simulink model "hexapod"  (R2022a)
settings: Solver=ode2  StartTime=0.0  StopTime=10.0  FixedStep=1e-4  RelTol=1e-3  AbsTol=1e-3  EnableMultiTasking=on
values from neighbouring files (symbols this model uses):
  N = 2    [gen_singleGait.m]
  s = t/T    [gait_mv_backward.m]    (also in gait_mv_forward.m; gait_mv_left.m; gait_mv_right.m; gait_rot_clockwise.m)
undefined symbols (not defined in the file or in its folder): X, Y, Z
libraries: sm_lib x90, nesl_utility x19, Contact_Forces_Lib x6, simulink x1
(part 1 of 4)
settings Model: Creator=world  LastModifiedBy=world
settings SolverCC: AutoScaleAbsTol=off  AlgebraicLoopSolver=TrustRegion  MaxZcPerStep=1
settings DataIOCC: LimitDataPoints=on  MaxDataPoints=10000
settings OptimizationCC: LifeSpan=inf
settings DebuggingCC: UnconnectedInputMsg=warning  UnconnectedOutputMsg=warning  UnconnectedLineMsg=warning  AllowSymbolicDim=off  SFUnexpectedBacktrackingDiag=warning  SFNoUnconditionalDefaultTransitionDiag=warning  SFExecutionAtInitializationDiag=none  SFMachineParentedDataDiag=warning  ArithmeticOperatorsInVariantConditions=warning
settings SFSimCC: SimUseLocalCustomCode=off  CustomCodeUndefinedFunction=UseInterfaceOnly
settings RTWCC: RTWUseLocalCustomCode=off  DLArmComputeVersion=19.05
settings CodeAppCC: StateflowObjectComments=on
settings GRTTargetCC: TargetLangStandard=C89/C90 (ANSI)
settings ConfigComp: CovMetricSettings=dw  CovSaveCumulativeToWorkspaceVar=on  CovSaveSingleToWorkspaceVar=on  CovExternalEMLEnable=off  CovSFcnEnable=off
settings SimscapeCC: SimscapeLogType=all  SimscapeLogSimulationStatistics=on  SimscapeLogDataHistory=10000
settings DiagnosticsConfigSet: SimMechanicsRigidlyBoundBlock=warning

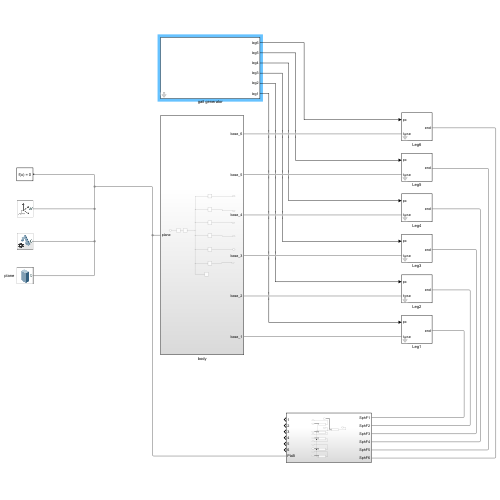
[thumbnail: Simulink's stored preview of the top-level diagram]
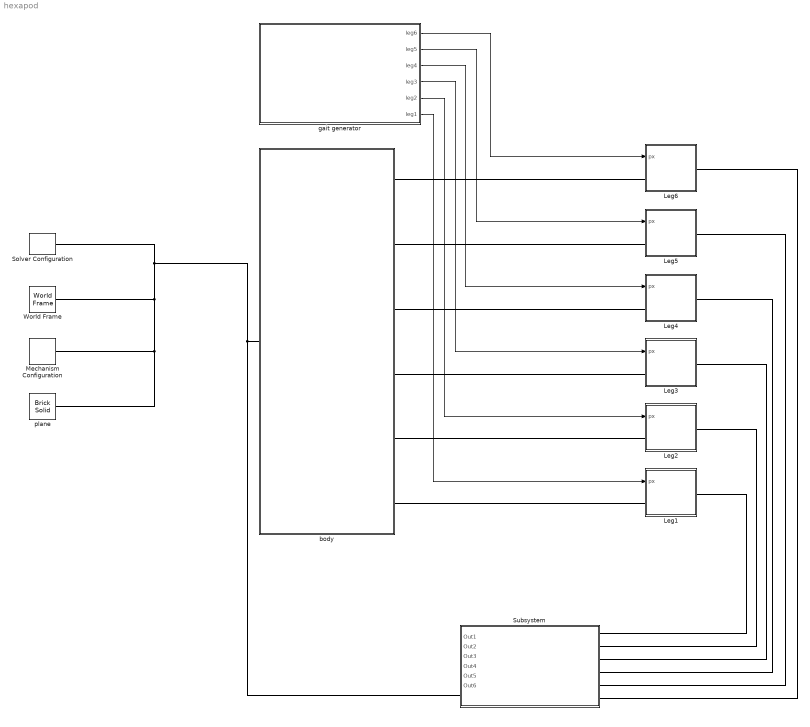
== system hexapod ==
  Leg1 : Subsystem  mask{LegNumber=1, theta1=80, theta2=90, theta3=100, l1=45, l2=93.5, l3=124.14, xx1=115, yy1=65, yy2=95}
      mask prompts: LegNumber "腿号"
      mask DialogControl ParameterGroupVar Prompt: 参数
  Leg2 : Subsystem  mask{LegNumber=2, theta1=80, theta2=90, theta3=100, l1=45, l2=93.5, l3=124.14, xx1=115, yy1=65, yy2=95}
      mask prompts: LegNumber "腿号"
      mask DialogControl ParameterGroupVar Prompt: 参数
  Leg3 : Subsystem  mask{LegNumber=3, theta1=80, theta2=90, theta3=100, l1=45, l2=93.5, l3=124.14, xx1=115, yy1=65, yy2=95}
      mask prompts: LegNumber "腿号"
      mask DialogControl ParameterGroupVar Prompt: 参数
  Leg4 : Subsystem  mask{LegNumber=4, theta1=80, theta2=90, theta3=100, l1=45, l2=93.5, l3=124.14, xx1=115, yy1=65, yy2=95}
      mask prompts: LegNumber "腿号"
      mask DialogControl ParameterGroupVar Prompt: 参数
  Leg5 : Subsystem  mask{LegNumber=5, theta1=80, theta2=90, theta3=100, l1=45, l2=93.5, l3=124.14, xx1=115, yy1=65, yy2=95}
      mask prompts: LegNumber "腿号"
      mask DialogControl ParameterGroupVar Prompt: 参数
  Leg6 : Subsystem  mask{LegNumber=6, theta1=80, theta2=90, theta3=100, l1=45, l2=93.5, l3=124.14, xx1=115, yy1=65, yy2=95}
      mask prompts: LegNumber "腿号"
      mask DialogControl ParameterGroupVar Prompt: 关键参数
      mask DialogControl Container4 Prompt: 几何参数
  Mechanism Configuration : sm_lib/Utilities/Mechanism Configuration  UniformGravity=Constant  GravityVector=[0 0 -9.80665]  GravityUnits=m/s^2  LinearizationDelta=0.001  JointModeTransitionNonlinearIterations=2
  Solver Configuration : nesl_utility/Solver Configuration  PhysicalDomain=network_engine_domain  SubClassName=solver  LeftPortType=input  RightPortType=generic  Tones=[]  Harmonics=[]  SimulateNoise=off  Profile=off  UseLocalSampling=off  EnableSwitchedLinearOptims=on  FrequencyDomain=off  UseCCode=off  RelTol=0.001  AbsTol=1e-06  MinStep=1e-09  ToWorkspace=off  RevertToSquareIcSolve=off  NumHomotopyIterations=100  PhasorMode=off  PhasorModeNumHarmonics=1  IndexReductionMethod=DerivativeReplacement  DoDC=off  ResidualTolerance=1e-09  UseLocalSolver=off  LocalSolverChoice=NE_BACKWARD_EULER_ADVANCER  LocalSolverSampleTime=0.001  DoFixedCost=off  MaxNonlinIter=3  MaxModeIter=2  ComputeImpulses=off  ImpulseIterations=2  LinearAlgebra=Sparse  LinearAlgebraNumThread=0  EquationFormulation=NE_TIME_EF  DelaysMemoryBudget=1024  AutomaticFiltering=on  FilteringTimeConstant=0.001  PartitionStorageMethod=AS_NEEDED  PartitionMemoryBudget=1024  PartitionMethod=FAST
      settings: SourceProductBaseCode=SS,PW,VE
  Subsystem : Subsystem
  World Frame : sm_lib/Frames and Transforms/World Frame
  body : Subsystem
  gait generator : Subsystem  mask{mode=high position, action=rotate clockwise, LL=2*50, AAng=45, HH=60, xx1=115, yy1=65, yy2=95, theta1=80, theta2=90, theta3=100, xxx1=[136.27,142.15], yyy1=[191.37,224.71], yyy2=[233.14,257], zzz1=[-67.38,-118]}
      mask TypeOptions mode: low position | high position
      mask TypeOptions action: move forward | move backward | move left | move right | rotate counterclockwise | rotate clockwise
      mask DialogControl Container6 Prompt: modification
      mask DialogControl Container7 Prompt: parameter
      mask DialogControl Container8 Prompt: gait parameter
      mask DialogControl Container5 Prompt: mechanical configuration
  plane : sm_lib/Body Elements/Brick Solid  GraphicAmbientColor=[0.15 0.15 0.15 1.0]  BasedOnType=Density  BrickDimensions=[5000 5000 1]  BrickDimensionUnits=mm  CenterOfMass=[0 0 0]  CenterOfMassUnits=m  GraphicDiffuseColor=[0.5 0.5 0.5]  Density=1000  DensityUnits=kg/m^3  DoExposeReferenceFrame=on  GraphicEmissiveColor=[0.0 0.0 0.0 1.0]  ExportEntireGeometry=off  SerializedFrames=<Frames/>  MarkerShape=Sphere  MarkerSize=10  GraphicType=FromGeometry  InertiaType=CalculateFromGeometry  Mass=1  MassUnits=kg  MomentsOfInertia=[1 1 1]  MomentsOfInertiaUnits=kg*m^2  GraphicOpacity=1.0  ProductsOfInertia=[0 0 0]  ProductsOfInertiaUnits=kg*m^2  GraphicShininess=75  GraphicSpecularColor=[0.5 0.5 0.5 1.0]  GraphicVisPropType=SimpleVisualProperties
  wires:
  gait generator/1(leg6) -> Leg6/1(px)
  gait generator/2(leg5) -> Leg5/1(px)
  gait generator/3(leg4) -> Leg4/1(px)
  gait generator/4(leg3) -> Leg3/1(px)
  gait generator/5(leg2) -> Leg2/1(px)
  gait generator/6(leg1) -> Leg1/1(px)
  connections:
  plane/RConn1 -- Mechanism Configuration/RConn1 -- World Frame/RConn1 -- Solver Configuration/RConn1 -- Subsystem/RConn1 -- body/LConn1
  Leg2/RConn1 -- Subsystem/LConn2
  Leg3/RConn1 -- Subsystem/LConn3
  Subsystem/LConn4 -- Leg4/RConn1
  Leg5/RConn1 -- Subsystem/LConn5
  Subsystem/LConn6 -- Leg6/RConn1
  Leg1/LConn1 -- body/RConn6
  Leg1/RConn1 -- Subsystem/LConn1
  body/RConn5 -- Leg2/LConn1
  body/RConn4 -- Leg3/LConn1
  body/RConn3 -- Leg4/LConn1
  Leg5/LConn1 -- body/RConn2
  body/RConn1 -- Leg6/LConn1

== system hexapod/Leg1 ==
  px : Inport
  Constant : Constant  Value=theta1
  Constant1 : Constant  Value=theta2
  Constant2 : Constant  Value=theta3
  Constant3 : Constant  Value=l1
  Constant4 : Constant  Value=l2
  Constant5 : Constant  Value=l3
  Constant6 : Constant  Value=xx1
  Constant7 : Constant  Value=yy1
  Constant8 : Constant  Value=yy2
  Demux : Demux  Outputs=3
  leg1 : Subsystem
  w-leg1 : Subsystem
  base : PMIOPort  Side=Left
  end : PMIOPort  Port=2  Side=Right
  wires:
  Constant8/1 -> w-leg1/12(yy2)
  Constant7/1 -> w-leg1/11(yy1)
  Constant6/1 -> w-leg1/10(xx1)
  Constant/1 -> w-leg1/4(theta1)
  Constant1/1 -> w-leg1/5(theta2)
  Constant2/1 -> w-leg1/6(theta3)
  Constant3/1 -> w-leg1/7(l1)
  Constant4/1 -> w-leg1/8(l2)
  Constant5/1 -> w-leg1/9(l3)
  Demux/1 -> w-leg1/1(x0)
  Demux/2 -> w-leg1/2(y0)
  Demux/3 -> w-leg1/3(z0)
  px/1 -> Demux/1
  connections:
  base/RConn1 -- leg1/LConn1
  leg1/RConn1 -- end/RConn1
  w-leg1/RConn3 -- leg1/LConn4
  leg1/LConn2 -- w-leg1/RConn1
  w-leg1/RConn2 -- leg1/LConn3

== system hexapod/Leg2 ==
  px : Inport
  Constant : Constant  Value=theta1
  Constant1 : Constant  Value=theta2
  Constant2 : Constant  Value=theta3
  Constant3 : Constant  Value=l1
  Constant4 : Constant  Value=l2
  Constant5 : Constant  Value=l3
  Constant6 : Constant  Value=xx1
  Constant7 : Constant  Value=yy1
  Constant8 : Constant  Value=yy2
  Demux : Demux  Outputs=3
  leg1 : Subsystem
  w-leg1 : Subsystem
  base : PMIOPort  Side=Left
  end : PMIOPort  Port=2  Side=Right
  wires:
  px/1 -> Demux/1
  Demux/3 -> w-leg1/3(z0)
  Demux/2 -> w-leg1/2(y0)
  Demux/1 -> w-leg1/1(x0)
  Constant5/1 -> w-leg1/9(l3)
  Constant4/1 -> w-leg1/8(l2)
  Constant3/1 -> w-leg1/7(l1)
  Constant2/1 -> w-leg1/6(theta3)
  Constant1/1 -> w-leg1/5(theta2)
  Constant/1 -> w-leg1/4(theta1)
  Constant6/1 -> w-leg1/10(xx1)
  Constant7/1 -> w-leg1/11(yy1)
  Constant8/1 -> w-leg1/12(yy2)
  connections:
  w-leg1/RConn2 -- leg1/LConn3
  leg1/LConn2 -- w-leg1/RConn1
  w-leg1/RConn3 -- leg1/LConn4
  leg1/RConn1 -- end/RConn1
  base/RConn1 -- leg1/LConn1

== system hexapod/Leg3 ==
  px : Inport
  Constant : Constant  Value=theta1
  Constant1 : Constant  Value=theta2
  Constant2 : Constant  Value=theta3
  Constant3 : Constant  Value=l1
  Constant4 : Constant  Value=l2
  Constant5 : Constant  Value=l3
  Constant6 : Constant  Value=xx1
  Constant7 : Constant  Value=yy1
  Constant8 : Constant  Value=yy2
  Demux : Demux  Outputs=3
  leg1 : Subsystem
  w-leg1 : Subsystem
  base : PMIOPort  Side=Left
  end : PMIOPort  Port=2  Side=Right
  wires:
  Constant8/1 -> w-leg1/12(yy2)
  Constant7/1 -> w-leg1/11(yy1)
  Constant6/1 -> w-leg1/10(xx1)
  Constant/1 -> w-leg1/4(theta1)
  Constant1/1 -> w-leg1/5(theta2)
  Constant2/1 -> w-leg1/6(theta3)
  Constant3/1 -> w-leg1/7(l1)
  Constant4/1 -> w-leg1/8(l2)
  Constant5/1 -> w-leg1/9(l3)
  Demux/1 -> w-leg1/1(x0)
  Demux/2 -> w-leg1/2(y0)
  Demux/3 -> w-leg1/3(z0)
  px/1 -> Demux/1
  connections:
  base/RConn1 -- leg1/LConn1
  leg1/RConn1 -- end/RConn1
  w-leg1/RConn3 -- leg1/LConn4
  leg1/LConn2 -- w-leg1/RConn1
  w-leg1/RConn2 -- leg1/LConn3

== system hexapod/Leg4 ==
  px : Inport
  Constant : Constant  Value=theta1
  Constant1 : Constant  Value=theta2
  Constant2 : Constant  Value=theta3
  Constant3 : Constant  Value=l1
  Constant4 : Constant  Value=l2
  Constant5 : Constant  Value=l3
  Constant6 : Constant  Value=xx1
  Constant7 : Constant  Value=yy1
  Constant8 : Constant  Value=yy2
  Demux : Demux  Outputs=3
  leg1 : Subsystem
  w-leg1 : Subsystem
  base : PMIOPort  Side=Left
  end : PMIOPort  Port=2  Side=Right
  wires:
  px/1 -> Demux/1
  Demux/3 -> w-leg1/3(z0)
  Demux/2 -> w-leg1/2(y0)
  Demux/1 -> w-leg1/1(x0)
  Constant5/1 -> w-leg1/9(l3)
  Constant4/1 -> w-leg1/8(l2)
  Constant3/1 -> w-leg1/7(l1)
  Constant2/1 -> w-leg1/6(theta3)
  Constant1/1 -> w-leg1/5(theta2)
  Constant/1 -> w-leg1/4(theta1)
  Constant6/1 -> w-leg1/10(xx1)
  Constant7/1 -> w-leg1/11(yy1)
  Constant8/1 -> w-leg1/12(yy2)
  connections:
  w-leg1/RConn2 -- leg1/LConn3
  leg1/LConn2 -- w-leg1/RConn1
  w-leg1/RConn3 -- leg1/LConn4
  leg1/RConn1 -- end/RConn1
  base/RConn1 -- leg1/LConn1

== system hexapod/Leg5 ==
  px : Inport
  Constant : Constant  Value=theta1
  Constant1 : Constant  Value=theta2
  Constant2 : Constant  Value=theta3
  Constant3 : Constant  Value=l1
  Constant4 : Constant  Value=l2
  Constant5 : Constant  Value=l3
  Constant6 : Constant  Value=xx1
  Constant7 : Constant  Value=yy1
  Constant8 : Constant  Value=yy2
  Demux : Demux  Outputs=3
  leg1 : Subsystem
  w-leg1 : Subsystem
  base : PMIOPort  Side=Left
  end : PMIOPort  Port=2  Side=Right
  wires:
  Constant8/1 -> w-leg1/12(yy2)
  Constant7/1 -> w-leg1/11(yy1)
  Constant6/1 -> w-leg1/10(xx1)
  Constant/1 -> w-leg1/4(theta1)
  Constant1/1 -> w-leg1/5(theta2)
  Constant2/1 -> w-leg1/6(theta3)
  Constant3/1 -> w-leg1/7(l1)
  Constant4/1 -> w-leg1/8(l2)
  Constant5/1 -> w-leg1/9(l3)
  Demux/1 -> w-leg1/1(x0)
  Demux/2 -> w-leg1/2(y0)
  Demux/3 -> w-leg1/3(z0)
  px/1 -> Demux/1
  connections:
  base/RConn1 -- leg1/LConn1
  leg1/RConn1 -- end/RConn1
  w-leg1/RConn3 -- leg1/LConn4
  leg1/LConn2 -- w-leg1/RConn1
  w-leg1/RConn2 -- leg1/LConn3

== system hexapod/Leg6 ==
  note: w-leg1
  px : Inport
  Constant : Constant  Value=theta1
  Constant1 : Constant  Value=theta2
  Constant2 : Constant  Value=theta3
  Constant3 : Constant  Value=l1
  Constant4 : Constant  Value=l2
  Constant5 : Constant  Value=l3
  Constant6 : Constant  Value=xx1
  Constant7 : Constant  Value=yy1
  Constant8 : Constant  Value=yy2
  Constant9 : Constant  Value=LegNumber
  Demux : Demux  Outputs=3
  MATLAB Function : MATLAB Function  TreatAsAtomicUnit=on
  Scope : Scope  NumInputPorts=3
  Scope1 : Scope  NumInputPorts=3
  Simulink-PS Converter : nesl_utility/Simulink-PS Converter  PhysicalDomain=network_engine_domain  SubClassName=ps_input  LeftPortType=input  RightPortType=output  PseudoPeriodic=off  Frequencies=[]  NoiseDistribution=none  NoiseParameters=[]  Unit=1  AffineConversion=off  FilteringAndDerivatives=filter  SimscapeFilterOrder=2  InputFilterTimeConstant=0.001  UdotUserProvided=0
      settings: SourceProductBaseCode=SS,PW,VE
  Simulink-PS Converter1 : nesl_utility/Simulink-PS Converter  PhysicalDomain=network_engine_domain  SubClassName=ps_input  LeftPortType=input  RightPortType=output  PseudoPeriodic=off  Frequencies=[]  NoiseDistribution=none  NoiseParameters=[]  Unit=1  AffineConversion=off  FilteringAndDerivatives=filter  SimscapeFilterOrder=2  InputFilterTimeConstant=0.001  UdotUserProvided=0
      settings: SourceProductBaseCode=SS,PW,VE
  Simulink-PS Converter2 : nesl_utility/Simulink-PS Converter  PhysicalDomain=network_engine_domain  SubClassName=ps_input  LeftPortType=input  RightPortType=output  PseudoPeriodic=off  Frequencies=[]  NoiseDistribution=none  NoiseParameters=[]  Unit=1  AffineConversion=off  FilteringAndDerivatives=filter  SimscapeFilterOrder=2  InputFilterTimeConstant=0.001  UdotUserProvided=0
      settings: SourceProductBaseCode=SS,PW,VE
  leg1 : Subsystem
  base : PMIOPort  Side=Left
  end : PMIOPort  Port=2  Side=Right
  wires:
  MATLAB Function/3(ang3) -> Simulink-PS Converter2/1, Scope/3
  px/1 -> Demux/1
  Demux/2 -> Scope1/2, MATLAB Function/3(y0)
  Demux/3 -> Scope1/3, MATLAB Function/4(z0)
  Demux/1 -> Scope1/1, MATLAB Function/2(x0)
  Constant9/1 -> MATLAB Function/1(i)
  MATLAB Function/2(ang2) -> Scope/2, Simulink-PS Converter1/1
  MATLAB Function/1(ang1) -> Scope/1, Simulink-PS Converter/1
  Constant2/1 -> MATLAB Function/7(theta3)
  Constant/1 -> MATLAB Function/5(theta1)
  Constant5/1 -> MATLAB Function/10(l3)
  Constant4/1 -> MATLAB Function/9(l2)
  Constant3/1 -> MATLAB Function/8(l1)
  Constant1/1 -> MATLAB Function/6(theta2)
  Constant6/1 -> MATLAB Function/11(xx1)
  Constant7/1 -> MATLAB Function/12(yy1)
  Constant8/1 -> MATLAB Function/13(yy2)
  connections:
  base/RConn1 -- leg1/LConn1
  leg1/RConn1 -- end/RConn1
  Simulink-PS Converter2/RConn1 -- leg1/LConn4
  Simulink-PS Converter/RConn1 -- leg1/LConn2
  Simulink-PS Converter1/RConn1 -- leg1/LConn3

== system hexapod/Subsystem ==
  Sphere to Plane Force{,1..5} (6 alike) : Contact_Forces_Lib/3D/Sphere to Plane Force  sphere_rad=0.01  plane_lenx=5  plane_leny=5  plane_depth=0.01  force_law=Linear  k_contact=1e7  b_contact=1e3  pen_full_damp_F=1e-4  pen_exponent=1  custom_param_1=1  custom_param_2=1  friction_law=Stick-Slip Continuous  mu_kinetic=0.5  mu_static=0.7  v_thr=0.001  vis_on=on  vis_opc_en=0  vis_len_plaBz=0.005  vis_clr=[0.9 0.2 0.2]  vis_opc=0.7
  SphF1 : PMIOPort  Side=Left
  SphF2 : PMIOPort  Port=2  Side=Left
  SphF3 : PMIOPort  Port=3  Side=Left
  PlaB : PMIOPort  Port=4  Side=Right
  SphF4 : PMIOPort  Port=5  Side=Left
  SphF5 : PMIOPort  Port=6  Side=Left
  SphF6 : PMIOPort  Port=7  Side=Left
  Out1 : Outport
  Out2 : Outport  Port=2
  Out3 : Outport  Port=3
  Out4 : Outport  Port=4
  Out5 : Outport  Port=5
  Out6 : Outport  Port=6
  wires:
  Sphere to Plane Force3/1 -> Out4/1
  Sphere to Plane Force1/1 -> Out2/1
  Sphere to Plane Force4/1 -> Out5/1
  Sphere to Plane Force5/1 -> Out6/1
  Sphere to Plane Force2/1 -> Out3/1
  Sphere to Plane Force/1 -> Out1/1
  connections:
  SphF3/RConn1 -- Sphere to Plane Force3/LConn1
  SphF1/RConn1 -- Sphere to Plane Force5/LConn1
  SphF4/RConn1 -- Sphere to Plane Force2/LConn1
  SphF2/RConn1 -- Sphere to Plane Force4/LConn1
  Sphere to Plane Force5/RConn1 -- Sphere to Plane Force/RConn1 -- Sphere to Plane Force3/RConn1 -- Sphere to Plane Force4/RConn1 -- Sphere to Plane Force2/RConn1 -- Sphere to Plane Force1/RConn1 -- PlaB/RConn1
  Sphere to Plane Force/LConn1 -- SphF6/RConn1
  SphF5/RConn1 -- Sphere to Plane Force1/LConn1

== system hexapod/body ==
  6-DOF Joint : sm_lib/Joints/6-DOF Joint  JointMode=Normal  SenseConstraintForce=off  SenseConstraintForceX=off  SenseConstraintForceY=off  SenseConstraintForceZ=off  SenseConstraintTorque=off  SenseConstraintTorqueX=off  SenseConstraintTorqueY=off  SenseConstraintTorqueZ=off  SenseTotalForce=off  SenseTotalForceX=off  SenseTotalForceY=off  SenseTotalForceZ=off  SenseTotalTorque=off  SenseTotalTorqueX=off  SenseTotalTorqueY=off  SenseTotalTorqueZ=off  CompositeWrenchDir=FollowerOnBase  CompositeWrenchFrame=BaseFrame  PxEquilibriumPosition=0  PxEquilibriumPositionUnits=m  PxSpringStiffness=0  PxSpringStiffnessUnits=N/m  PxDampingCoefficient=0  PxDampingCoefficientUnits=N/(m/s)  PxTorqueActuationMode=NoTorque  PxMotionActuationMode=ComputedMotion  PxSensePosition=off  PxSenseVelocity=off  PxSenseAcceleration=off  PxSenseTorqueForce=off  PxSenseLowerLimitTorqueForce=off  PxSenseUpperLimitTorqueForce=off  PxLowerLimitSpecify=off  PxLowerLimitBound=-1  PxLowerLimitBoundUnits=m  PxLowerLimitStiffness=1e6  PxLowerLimitStiffnessUnits=N/m  PxLowerLimitDamping=1e3  PxLowerLimitDampingUnits=N/(m/s)  PxLowerLimitTransitionRegionWidth=1e-4  PxLowerLimitTransitionRegionWidthUnits=m  PxUpperLimitSpecify=off  PxUpperLimitBound=1  PxUpperLimitBoundUnits=m  PxUpperLimitStiffness=1e6  PxUpperLimitStiffnessUnits=N/m  PxUpperLimitDamping=1e3  PxUpperLimitDampingUnits=N/(m/s)  PxUpperLimitTransitionRegionWidth=1e-4  PxUpperLimitTransitionRegionWidthUnits=m  PxPositionTargetSpecify=off  PxPositionTargetPriority=High  PxPositionTargetValue=0  PxPositionTargetValueUnits=m  PxVelocityTargetSpecify=off  PxVelocityTargetPriority=High  PxVelocityTargetValue=0  PxVelocityTargetValueUnits=m/s  PyEquilibriumPosition=0  PyEquilibriumPositionUnits=m  PySpringStiffness=0  PySpringStiffnessUnits=N/m  PyDampingCoefficient=0  PyDampingCoefficientUnits=N/(m/s)  PyTorqueActuationMode=NoTorque  PyMotionActuationMode=ComputedMotion  PySensePosition=off  PySenseVelocity=off  PySenseAcceleration=off  PySenseTorqueForce=off  PySenseLowerLimitTorqueForce=off  PySenseUpperLimitTorqueForce=off  PyLowerLimitSpecify=off  PyLowerLimitBound=-1  PyLowerLimitBoundUnits=m  PyLowerLimitStiffness=1e6  PyLowerLimitStiffnessUnits=N/m  PyLowerLimitDamping=1e3  PyLowerLimitDampingUnits=N/(m/s)  PyLowerLimitTransitionRegionWidth=1e-4  PyLowerLimitTransitionRegionWidthUnits=m  PyUpperLimitSpecify=off  PyUpperLimitBound=1  PyUpperLimitBoundUnits=m  PyUpperLimitStiffness=1e6  PyUpperLimitStiffnessUnits=N/m  PyUpperLimitDamping=1e3  PyUpperLimitDampingUnits=N/(m/s)  PyUpperLimitTransitionRegionWidth=1e-4  PyUpperLimitTransitionRegionWidthUnits=m  PyPositionTargetSpecify=off  PyPositionTargetPriority=High  PyPositionTargetValue=0  PyPositionTargetValueUnits=m  PyVelocityTargetSpecify=off  PyVelocityTargetPriority=High  PyVelocityTargetValue=0  PyVelocityTargetValueUnits=m/s  PzEquilibriumPosition=0  PzEquilibriumPositionUnits=m  PzSpringStiffness=0  PzSpringStiffnessUnits=N/m  PzDampingCoefficient=0  PzDampingCoefficientUnits=N/(m/s)  PzTorqueActuationMode=NoTorque  PzMotionActuationMode=ComputedMotion  PzSensePosition=off  PzSenseVelocity=off  PzSenseAcceleration=off  PzSenseTorqueForce=off  PzSenseLowerLimitTorqueForce=off  PzSenseUpperLimitTorqueForce=off  PzLowerLimitSpecify=off  PzLowerLimitBound=-1  PzLowerLimitBoundUnits=m  PzLowerLimitStiffness=1e6  PzLowerLimitStiffnessUnits=N/m  PzLowerLimitDamping=1e3  PzLowerLimitDampingUnits=N/(m/s)  PzLowerLimitTransitionRegionWidth=1e-4  PzLowerLimitTransitionRegionWidthUnits=m  PzUpperLimitSpecify=off  PzUpperLimitBound=1  PzUpperLimitBoundUnits=m  PzUpperLimitStiffness=1e6  PzUpperLimitStiffnessUnits=N/m  PzUpperLimitDamping=1e3  PzUpperLimitDampingUnits=N/(m/s)  PzUpperLimitTransitionRegionWidth=1e-4  PzUpperLimitTransitionRegionWidthUnits=m  PzPositionTargetSpecify=off  PzPositionTargetPriority=High  PzPositionTargetValue=0  PzPositionTargetValueUnits=m  PzVelocityTargetSpecify=off  PzVelocityTargetPriority=High  PzVelocityTargetValue=0  PzVelocityTargetValueUnits=m/s  SphDefPosRotationMethod=None  SphDefPosRotationAngleUnits=deg  SphDefPosRotationStandardAxis=+Z  SphDefPosRotationAngle=0.0  SphDefPosRotationArbitraryAxis=[0 0 1]  SphDefPosFollAlignAxisA=+X  SphDefPosBaseAlignAxisA=+Y  SphDefPosFollAlignAxisB=+Y  SphDefPosBaseAlignAxisB=+Z  SphDefPosRotationSequenceAxes=FollowerAxes  SphDefPosRotationSequence=XYX  SphDefPosRotationSequenceAngles=[0 0 0]  SphDefPosRotationSequenceAnglesUnits=deg  SphDefPosRotationMatrix=[1 0 0; 0 1 0; 0 0 1]  SphEqPosRotationMethod=None  SphEqPosRotationAngleUnits=deg  SphEqPosRotationStandardAxis=+Z  SphEqPosRotationAngle=0.0  SphEqPosRotationArbitraryAxis=[0 0 1]  SphEqPosFollAlignAxisA=+X  SphEqPosBaseAlignAxisA=+Y  SphEqPosFollAlignAxisB=+Y  SphEqPosBaseAlignAxisB=+Z  SphEqPosRotationSequenceAxes=FollowerAxes  SphEqPosRotationSequence=XYX  SphEqPosRotationSequenceAngles=[0 0 0]  SphEqPosRotationSequenceAnglesUnits=deg  SphEqPosRotationMatrix=[1 0 0; 0 1 0; 0 0 1]  SphSpringStiffness=0  SphSpringStiffnessUnits=N*m/deg  SphDampingCoefficient=0  SphDampingCoefficientUnits=N*m/(deg/s)  SphActuateTorqueX=off  SphActuateTorqueY=off  SphActuateTorqueZ=off  SphActuateTorque=off  SphTorqueActuationMode=NoTorque  SphMotionActuationMode=ComputedMotion  SphActuationFrame=BaseFrame  SphSensePosition=off  SphSenseVelocityX=off  SphSenseVelocityY=off  SphSenseVelocityZ=off  SphSenseVelocity=off  SphSenseAccelerationX=off  SphSenseAccelerationY=off  SphSenseAccelerationZ=off  SphSenseAcceleration=off  SphSenseTorqueX=off  SphSenseTorqueY=off  SphSenseTorqueZ=off  SphSenseTorqueForce=off  SphSenseLowerLimitTorqueMag=off  SphSenseUpperLimitTorqueMag=off  SphSensingFrame=BaseFrame  SphLowerLimitSpecify=off  SphLowerLimitBound=15  SphLowerLimitBoundUnits=deg  SphLowerLimitStiffness=1e4  SphLowerLimitStiffnessUnits=N*m/deg  SphLowerLimitDamping=10  SphLowerLimitDampingUnits=N*m/(deg/s)  SphLowerLimitTransitionRegionWidth=0.1  SphLowerLimitTransitionRegionWidthUnits=deg  SphUpperLimitSpecify=off  SphUpperLimitBound=45  SphUpperLimitBoundUnits=deg  SphUpperLimitStiffness=1e4  SphUpperLimitStiffnessUnits=N*m/deg  SphUpperLimitDamping=10  SphUpperLimitDampingUnits=N*m/(deg/s)  SphUpperLimitTransitionRegionWidth=0.1  SphUpperLimitTransitionRegionWidthUnits=deg  SphPositionTargetRotationMethod=None  SphPositionTargetRotationAngleUnits=deg  SphPositionTargetRotationStandardAxis=+Z  SphPositionTargetRotationAngle=0.0  SphPositionTargetRotationArbitraryAxis=[0 0 1]  SphPositionTargetFollAlignAxisA=+X  SphPositionTargetBaseAlignAxisA=+Y  SphPositionTargetFollAlignAxisB=+Y  SphPositionTargetBaseAlignAxisB=+Z  SphPositionTargetRotationSequenceAxes=FollowerAxes  SphPositionTargetRotationSequence=XYX  SphPositionTargetRotationSequenceAngles=[0 0 0]  SphPositionTargetRotationSequenceAnglesUnits=deg  SphPositionTargetRotationMatrix=[1 0 0; 0 1 0; 0 0 1]  SphPositionTargetSpecify=off  SphPositionTargetPriority=High  SphVelocityTargetValue=[0 0 0]  SphVelocityTargetValueUnits=deg/s  SphVelocityTargetSpecify=off  SphVelocityTargetPriority=High  SphVelocityTargetInFollowerFrame=on
  base1 : sm_lib/Frames and Transforms/Rigid Transform  TranslationMethod=Cartesian  TranslationStandardOffset=0  TranslationLengthUnit=mm  TranslationStandardAxis=+Z  TranslationCartesianOffset=[80.31 -61.58 0]  TranslationROffset=0  TranslationROffsetUnits=m  TranslationZOffset=0  TranslationZOffsetUnits=m  TranslationThetaOffset=0  TranslationThetaOffsetUnits=deg  RotationMethod=StandardAxis  RotationAngleUnits=deg  RotationStandardAxis=+Z  RotationAngle=-37.48  RotationArbitraryAxis=[0 0 1]  FollAlignAxisA=+X  BaseAlignAxisA=+Y  FollAlignAxisB=+Y  BaseAlignAxisB=+Z  RotationSequenceAxes=FollowerAxes  RotationSequence=XYX  RotationSequenceAngles=[0 0 0]  RotationSequenceAnglesUnits=deg  RotationMatrix=[1 0 0; 0 1 0; 0 0 1]
  base2 : sm_lib/Frames and Transforms/Rigid Transform  TranslationMethod=Cartesian  TranslationStandardOffset=0  TranslationLengthUnit=mm  TranslationStandardAxis=+Z  TranslationCartesianOffset=[0 93.7 0]  TranslationROffset=0  TranslationROffsetUnits=m  TranslationZOffset=0  TranslationZOffsetUnits=m  TranslationThetaOffset=0  TranslationThetaOffsetUnits=deg  RotationMethod=StandardAxis  RotationAngleUnits=deg  RotationStandardAxis=+Z  RotationAngle=90  RotationArbitraryAxis=[0 0 1]  FollAlignAxisA=+X  BaseAlignAxisA=+Y  FollAlignAxisB=+Y  BaseAlignAxisB=+Z  RotationSequenceAxes=FollowerAxes  RotationSequence=XYX  RotationSequenceAngles=[0 0 0]  RotationSequenceAnglesUnits=deg  RotationMatrix=[1 0 0; 0 1 0; 0 0 1]
  base3 : sm_lib/Frames and Transforms/Rigid Transform  TranslationMethod=Cartesian  TranslationStandardOffset=0  TranslationLengthUnit=mm  TranslationStandardAxis=+Z  TranslationCartesianOffset=[-80.31 -61.58 0]  TranslationROffset=0  TranslationROffsetUnits=m  TranslationZOffset=0  TranslationZOffsetUnits=m  TranslationThetaOffset=0  TranslationThetaOffsetUnits=deg  RotationMethod=StandardAxis  RotationAngleUnits=deg  RotationStandardAxis=+Z  RotationAngle=-142.52  RotationArbitraryAxis=[0 0 1]  FollAlignAxisA=+X  BaseAlignAxisA=+Y  FollAlignAxisB=+Y  BaseAlignAxisB=+Z  RotationSequenceAxes=FollowerAxes  RotationSequence=XYX  RotationSequenceAngles=[0 0 0]  RotationSequenceAnglesUnits=deg  RotationMatrix=[1 0 0; 0 1 0; 0 0 1]
  base4 : sm_lib/Frames and Transforms/Rigid Transform  TranslationMethod=Cartesian  TranslationStandardOffset=0  TranslationLengthUnit=mm  TranslationStandardAxis=+Z  TranslationCartesianOffset=[80.31 61.58 0]  TranslationROffset=0  TranslationROffsetUnits=m  TranslationZOffset=0  TranslationZOffsetUnits=m  TranslationThetaOffset=0  TranslationThetaOffsetUnits=deg  RotationMethod=StandardAxis  RotationAngleUnits=deg  RotationStandardAxis=+Z  RotationAngle=37.48  RotationArbitraryAxis=[0 0 1]  FollAlignAxisA=+X  BaseAlignAxisA=+Y  FollAlignAxisB=+Y  BaseAlignAxisB=+Z  RotationSequenceAxes=FollowerAxes  RotationSequence=XYX  RotationSequenceAngles=[0 0 0]  RotationSequenceAnglesUnits=deg  RotationMatrix=[1 0 0; 0 1 0; 0 0 1]
  base5 : sm_lib/Frames and Transforms/Rigid Transform  TranslationMethod=Cartesian  TranslationStandardOffset=0  TranslationLengthUnit=mm  TranslationStandardAxis=+Z  TranslationCartesianOffset=[0 -93.7 0]  TranslationROffset=0  TranslationROffsetUnits=m  TranslationZOffset=0  TranslationZOffsetUnits=m  TranslationThetaOffset=0  TranslationThetaOffsetUnits=deg  RotationMethod=StandardAxis  RotationAngleUnits=deg  RotationStandardAxis=+Z  RotationAngle=-90  RotationArbitraryAxis=[0 0 1]  FollAlignAxisA=+X  BaseAlignAxisA=+Y  FollAlignAxisB=+Y  BaseAlignAxisB=+Z  RotationSequenceAxes=FollowerAxes  RotationSequence=XYX  RotationSequenceAngles=[0 0 0]  RotationSequenceAnglesUnits=deg  RotationMatrix=[1 0 0; 0 1 0; 0 0 1]
  base6 : sm_lib/Frames and Transforms/Rigid Transform  TranslationMethod=Cartesian  TranslationStandardOffset=0  TranslationLengthUnit=mm  TranslationStandardAxis=+Z  TranslationCartesianOffset=[-80.31 61.58 0]  TranslationROffset=0  TranslationROffsetUnits=m  TranslationZOffset=0  TranslationZOffsetUnits=m  TranslationThetaOffset=0  TranslationThetaOffsetUnits=deg  RotationMethod=StandardAxis  RotationAngleUnits=deg  RotationStandardAxis=+Z  RotationAngle=142.52  RotationArbitraryAxis=[0 0 1]  FollAlignAxisA=+X  BaseAlignAxisA=+Y  FollAlignAxisB=+Y  BaseAlignAxisB=+Z  RotationSequenceAxes=FollowerAxes  RotationSequence=XYX  RotationSequenceAngles=[0 0 0]  RotationSequenceAnglesUnits=deg  RotationMatrix=[1 0 0; 0 1 0; 0 0 1]
  body : sm_lib/Body Elements/Brick Solid  GraphicAmbientColor=[0.15 0.15 0.15 1.0]  BasedOnType=Density  BrickDimensions=[215 61.45*2 20]  BrickDimensionUnits=mm  CenterOfMass=[0 0 0]  CenterOfMassUnits=m  GraphicDiffuseColor=[0.5 0.5 0.5]  Density=1000  DensityUnits=kg/m^3  DoExposeReferenceFrame=on  GraphicEmissiveColor=[0.0 0.0 0.0 1.0]  ExportEntireGeometry=off  SerializedFrames=<Frames/>  MarkerShape=Sphere  MarkerSize=10  GraphicType=FromGeometry  InertiaType=CalculateFromGeometry  Mass=1  MassUnits=kg  MomentsOfInertia=[1 1 1]  MomentsOfInertiaUnits=kg*m^2  GraphicOpacity=1.0  ProductsOfInertia=[0 0 0]  ProductsOfInertiaUnits=kg*m^2  GraphicShininess=75  GraphicSpecularColor=[0.5 0.5 0.5 1.0]  GraphicVisPropType=SimpleVisualProperties
  world : sm_lib/Frames and Transforms/Rigid Transform  TranslationMethod=Cartesian  TranslationStandardOffset=0  TranslationLengthUnit=mm  TranslationStandardAxis=+Z  TranslationCartesianOffset=[0 0 150]  TranslationROffset=0  TranslationROffsetUnits=m  TranslationZOffset=0  TranslationZOffsetUnits=m  TranslationThetaOffset=0  TranslationThetaOffsetUnits=deg  RotationMethod=None  RotationAngleUnits=deg  RotationStandardAxis=+Z  RotationAngle=0.0  RotationArbitraryAxis=[0 0 1]  FollAlignAxisA=+X  BaseAlignAxisA=+Y  FollAlignAxisB=+Y  BaseAlignAxisB=+Z  RotationSequenceAxes=FollowerAxes  RotationSequence=XYX  RotationSequenceAngles=[0 0 0]  RotationSequenceAnglesUnits=deg  RotationMatrix=[1 0 0; 0 1 0; 0 0 1]
  base_6 : PMIOPort  Side=Right
  base_5 : PMIOPort  Port=2  Side=Right
  base_4 : PMIOPort  Port=3  Side=Right
  plane : PMIOPort  Port=4  Side=Left
  base_3 : PMIOPort  Port=5  Side=Right
  base_2 : PMIOPort  Port=6  Side=Right
  base_1 : PMIOPort  Port=7  Side=Right
  connections:
  world/RConn1 -- base4/LConn1 -- base6/LConn1 -- base5/LConn1 -- base3/LConn1 -- base1/LConn1 -- body/RConn1 -- base2/LConn1
  base5/RConn1 -- base_5/RConn1
  base3/RConn1 -- base_3/RConn1
  6-DOF Joint/LConn1 -- plane/RConn1
  world/LConn1 -- 6-DOF Joint/RConn1
  base4/RConn1 -- base_4/RConn1
  base1/RConn1 -- base_1/RConn1
  base2/RConn1 -- base_2/RConn1
  base6/RConn1 -- base_6/RConn1

== system hexapod/gait generator ==
  Constant : Constant  Value=action
  If : If  IfExpression=u1 == 1  ElseIfExpressions=u1==2,u1==3,u1==4,u1==5,u1==6  ShowElse=off
  MergeLeg{1..6} (6 alike) : Merge  Inputs=6
  前进步态 : Subsystem  mask{xxx1=xxx1(mode), yyy1=yyy1(mode), yyy2=yyy2(mode), zzz1=zzz1(mode)}
      mask DialogControl ParameterGroupVar Prompt: 参数
  右移步态 : Subsystem  mask{xxx1=xxx1(mode), yyy1=yyy1(mode), yyy2=yyy2(mode), zzz1=zzz1(mode)}
      mask DialogControl ParameterGroupVar Prompt: 参数
  后退步态 : Subsystem  mask{xxx1=xxx1(mode), yyy1=yyy1(mode), yyy2=yyy2(mode), zzz1=zzz1(mode)}
      mask DialogControl ParameterGroupVar Prompt: 参数
  左移步态 : Subsystem  mask{xxx1=xxx1(mode), yyy1=yyy1(mode), yyy2=yyy2(mode), zzz1=zzz1(mode)}
      mask DialogControl ParameterGroupVar Prompt: 参数
  足尖轨迹生成 : Subsystem  mask{L=LL, H=HH}
      mask prompts: L "L（2*前进步长）"; H "H（抬腿高度）"
      mask DialogControl ParameterGroupVar Prompt: 参数
  逆时针旋转步态 : Subsystem  mask{xxx1=xxx1(mode), yyy1=yyy1(mode), yyy2=yyy2(mode), zzz1=zzz1(mode), theta1=theta1, theta2=theta2, theta3=theta3, Ang=AAng}
      mask DialogControl ParameterGroupVar Prompt: 参数
  顺时针旋转步态 : Subsystem  mask{xxx1=xxx1(mode), yyy1=yyy1(mode), yyy2=yyy2(mode), zzz1=zzz1(mode), theta1=theta1, theta2=theta2, theta3=theta3, Ang=AAng}
      mask DialogControl ParameterGroupVar Prompt: 参数
  leg6 : Outport
  leg5 : Outport  Port=2
  leg4 : Outport  Port=3
  leg3 : Outport  Port=4
  leg2 : Outport  Port=5
  leg1 : Outport  Port=6
  wires:
  MergeLeg6/1 -> leg6/1
  MergeLeg5/1 -> leg5/1
  逆时针旋转步态/2(Out2) -> MergeLeg2/6
  顺时针旋转步态/5(Out5) -> MergeLeg5/5
  逆时针旋转步态/5(Out5) -> MergeLeg5/6
  顺时针旋转步态/3(Out3) -> MergeLeg3/5
  顺时针旋转步态/2(Out2) -> MergeLeg2/5
  MergeLeg4/1 -> leg4/1
  后退步态/5(Out5) -> MergeLeg5/2
  左移步态/1(Out1) -> MergeLeg1/3
  右移步态/4(Out4) -> MergeLeg4/4
  If/4 -> 右移步态/Action
  逆时针旋转步态/3(Out3) -> MergeLeg3/6
  MergeLeg1/1 -> leg1/1
  MergeLeg3/1 -> leg3/1
  右移步态/2(Out2) -> MergeLeg2/4
  前进步态/2(Out2) -> MergeLeg2/1
  If/6 -> 逆时针旋转步态/Action
  右移步态/5(Out5) -> MergeLeg5/4
  左移步态/2(Out2) -> MergeLeg2/3
  左移步态/5(Out5) -> MergeLeg5/3
  左移步态/6(Out6) -> MergeLeg6/3
  前进步态/5(Out5) -> MergeLeg5/1
  右移步态/3(Out3) -> MergeLeg3/4
  顺时针旋转步态/6(Out6) -> MergeLeg6/5
  顺时针旋转步态/1(Out1) -> MergeLeg1/5
  左移步态/4(Out4) -> MergeLeg4/3
  逆时针旋转步态/1(Out1) -> MergeLeg1/6
  后退步态/4(Out4) -> MergeLeg4/2
  If/5 -> 顺时针旋转步态/Action
  If/3 -> 左移步态/Action
  前进步态/3(Out3) -> MergeLeg3/1
  MergeLeg2/1 -> leg2/1
  左移步态/3(Out3) -> MergeLeg3/3
  后退步态/3(Out3) -> MergeLeg3/2
  If/1 -> 前进步态/Action
  If/2 -> 后退步态/Action
  足尖轨迹生成/1(x1) -> 右移步态/1(x1), 左移步态/1(x1), 前进步态/1(x1), 后退步态/1(x1), 顺时针旋转步态/1(x1), 逆时针旋转步态/1(x1)
  右移步态/6(Out6) -> MergeLeg6/4
  前进步态/4(Out4) -> MergeLeg4/1
  前进步态/6(Out6) -> MergeLeg6/1
  后退步态/1(Out1) -> MergeLeg1/2
  顺时针旋转步态/4(Out4) -> MergeLeg4/5
  右移步态/1(Out1) -> MergeLeg1/4
  足尖轨迹生成/2(x2) -> 顺时针旋转步态/2(x2), 左移步态/2(x2), 前进步态/2(x2), 后退步态/2(x2), 右移步态/2(x2), 逆时针旋转步态/2(x2)
  后退步态/6(Out6) -> MergeLeg6/2
  逆时针旋转步态/4(Out4) -> MergeLeg4/6
  前进步态/1(Out1) -> MergeLeg1/1
  后退步态/2(Out2) -> MergeLeg2/2
  足尖轨迹生成/5(LL) -> 顺时针旋转步态/5(LL0), 逆时针旋转步态/5(LL0)
  足尖轨迹生成/4(z2) -> 右移步态/4(z2), 左移步态/4(z2), 前进步态/4(z2), 后退步态/4(z2), 顺时针旋转步态/4(z2), 逆时针旋转步态/4(z2)
  逆时针旋转步态/6(Out6) -> MergeLeg6/6
  足尖轨迹生成/3(z1) -> 左移步态/3(z1), 前进步态/3(z1), 后退步态/3(z1), 右移步态/3(z1), 顺时针旋转步态/3(z1), 逆时针旋转步态/3(z1)
  Constant/1 -> If/1

== system hexapod/Leg1/leg1 ==
  Revolute Joint : sm_lib/Joints/Revolute Joint  JointMode=Normal  SenseConstraintForce=off  SenseConstraintForceX=off  SenseConstraintForceY=off  SenseConstraintForceZ=off  SenseConstraintTorque=off  SenseConstraintTorqueX=off  SenseConstraintTorqueY=off  SenseConstraintTorqueZ=off  SenseTotalForce=off  SenseTotalForceX=off  SenseTotalForceY=off  SenseTotalForceZ=off  SenseTotalTorque=off  SenseTotalTorqueX=off  SenseTotalTorqueY=off  SenseTotalTorqueZ=off  CompositeWrenchDir=FollowerOnBase  CompositeWrenchFrame=BaseFrame  EquilibriumPosition=0  EquilibriumPositionUnits=deg  SpringStiffness=0  SpringStiffnessUnits=N*m/deg  DampingCoefficient=0  DampingCoefficientUnits=N*m/(deg/s)  TorqueActuationMode=ComputedTorque  MotionActuationMode=InputMotion  SensePosition=off  SenseVelocity=off  SenseAcceleration=off  SenseTorqueForce=off  SenseLowerLimitTorqueForce=off  SenseUpperLimitTorqueForce=off  LowerLimitSpecify=off  LowerLimitBound=-90  LowerLimitBoundUnits=deg  LowerLimitStiffness=1e4  LowerLimitStiffnessUnits=N*m/deg  LowerLimitDamping=10  LowerLimitDampingUnits=N*m/(deg/s)  LowerLimitTransitionRegionWidth=0.1  LowerLimitTransitionRegionWidthUnits=deg  UpperLimitSpecify=off  UpperLimitBound=90  UpperLimitBoundUnits=deg  UpperLimitStiffness=1e4  UpperLimitStiffnessUnits=N*m/deg  UpperLimitDamping=10  UpperLimitDampingUnits=N*m/(deg/s)  UpperLimitTransitionRegionWidth=0.1  UpperLimitTransitionRegionWidthUnits=deg  PositionTargetSpecify=off  PositionTargetPriority=High  PositionTargetValue=0  PositionTargetValueUnits=deg  VelocityTargetSpecify=off  VelocityTargetPriority=High  VelocityTargetValue=0  VelocityTargetValueUnits=deg/s
  Revolute Joint1 : sm_lib/Joints/Revolute Joint  JointMode=Normal  SenseConstraintForce=off  SenseConstraintForceX=off  SenseConstraintForceY=off  SenseConstraintForceZ=off  SenseConstraintTorque=off  SenseConstraintTorqueX=off  SenseConstraintTorqueY=off  SenseConstraintTorqueZ=off  SenseTotalForce=off  SenseTotalForceX=off  SenseTotalForceY=off  SenseTotalForceZ=off  SenseTotalTorque=off  SenseTotalTorqueX=off  SenseTotalTorqueY=off  SenseTotalTorqueZ=off  CompositeWrenchDir=FollowerOnBase  CompositeWrenchFrame=BaseFrame  EquilibriumPosition=0  EquilibriumPositionUnits=deg  SpringStiffness=0  SpringStiffnessUnits=N*m/deg  DampingCoefficient=0  DampingCoefficientUnits=N*m/(deg/s)  TorqueActuationMode=ComputedTorque  MotionActuationMode=InputMotion  SensePosition=off  SenseVelocity=off  SenseAcceleration=off  SenseTorqueForce=off  SenseLowerLimitTorqueForce=off  SenseUpperLimitTorqueForce=off  LowerLimitSpecify=off  LowerLimitBound=-90  LowerLimitBoundUnits=deg  LowerLimitStiffness=1e4  LowerLimitStiffnessUnits=N*m/deg  LowerLimitDamping=10  LowerLimitDampingUnits=N*m/(deg/s)  LowerLimitTransitionRegionWidth=0.1  LowerLimitTransitionRegionWidthUnits=deg  UpperLimitSpecify=off  UpperLimitBound=90  UpperLimitBoundUnits=deg  UpperLimitStiffness=1e4  UpperLimitStiffnessUnits=N*m/deg  UpperLimitDamping=10  UpperLimitDampingUnits=N*m/(deg/s)  UpperLimitTransitionRegionWidth=0.1  UpperLimitTransitionRegionWidthUnits=deg  PositionTargetSpecify=off  PositionTargetPriority=High  PositionTargetValue=0  PositionTargetValueUnits=deg  VelocityTargetSpecify=off  VelocityTargetPriority=High  VelocityTargetValue=0  VelocityTargetValueUnits=deg/s
  Revolute Joint2 : sm_lib/Joints/Revolute Joint  JointMode=Normal  SenseConstraintForce=off  SenseConstraintForceX=off  SenseConstraintForceY=off  SenseConstraintForceZ=off  SenseConstraintTorque=off  SenseConstraintTorqueX=off  SenseConstraintTorqueY=off  SenseConstraintTorqueZ=off  SenseTotalForce=off  SenseTotalForceX=off  SenseTotalForceY=off  SenseTotalForceZ=off  SenseTotalTorque=off  SenseTotalTorqueX=off  SenseTotalTorqueY=off  SenseTotalTorqueZ=off  CompositeWrenchDir=FollowerOnBase  CompositeWrenchFrame=BaseFrame  EquilibriumPosition=0  EquilibriumPositionUnits=deg  SpringStiffness=0  SpringStiffnessUnits=N*m/deg  DampingCoefficient=0  DampingCoefficientUnits=N*m/(deg/s)  TorqueActuationMode=ComputedTorque  MotionActuationMode=InputMotion  SensePosition=off  SenseVelocity=off  SenseAcceleration=off  SenseTorqueForce=off  SenseLowerLimitTorqueForce=off  SenseUpperLimitTorqueForce=off  LowerLimitSpecify=off  LowerLimitBound=-90  LowerLimitBoundUnits=deg  LowerLimitStiffness=1e4  LowerLimitStiffnessUnits=N*m/deg  LowerLimitDamping=10  LowerLimitDampingUnits=N*m/(deg/s)  LowerLimitTransitionRegionWidth=0.1  LowerLimitTransitionRegionWidthUnits=deg  UpperLimitSpecify=off  UpperLimitBound=90  UpperLimitBoundUnits=deg  UpperLimitStiffness=1e4  UpperLimitStiffnessUnits=N*m/deg  UpperLimitDamping=10  UpperLimitDampingUnits=N*m/(deg/s)  UpperLimitTransitionRegionWidth=0.1  UpperLimitTransitionRegionWidthUnits=deg  PositionTargetSpecify=off  PositionTargetPriority=High  PositionTargetValue=0  PositionTargetValueUnits=deg  VelocityTargetSpecify=off  VelocityTargetPriority=High  VelocityTargetValue=0  VelocityTargetValueUnits=deg/s
  link1 : Subsystem
  link2 : Subsystem
  link3 : Subsystem
  base : PMIOPort  Side=Left
  ang1 : PMIOPort  Port=2  Side=Left
  ang2 : PMIOPort  Port=3  Side=Left
  ang3 : PMIOPort  Port=4  Side=Left
  end : PMIOPort  Port=5  Side=Right
  connections:
  Revolute Joint2/LConn2 -- ang3/RConn1
  Revolute Joint/LConn2 -- ang1/RConn1
  Revolute Joint/RConn1 -- link1/LConn1
  Revolute Joint2/RConn1 -- link3/LConn1
  Revolute Joint1/LConn1 -- link1/RConn1
  link2/LConn1 -- Revolute Joint1/RConn1
  Revolute Joint2/LConn1 -- link2/RConn1
  end/RConn1 -- link3/RConn1
  base/RConn1 -- Revolute Joint/LConn1
  Revolute Joint1/LConn2 -- ang2/RConn1

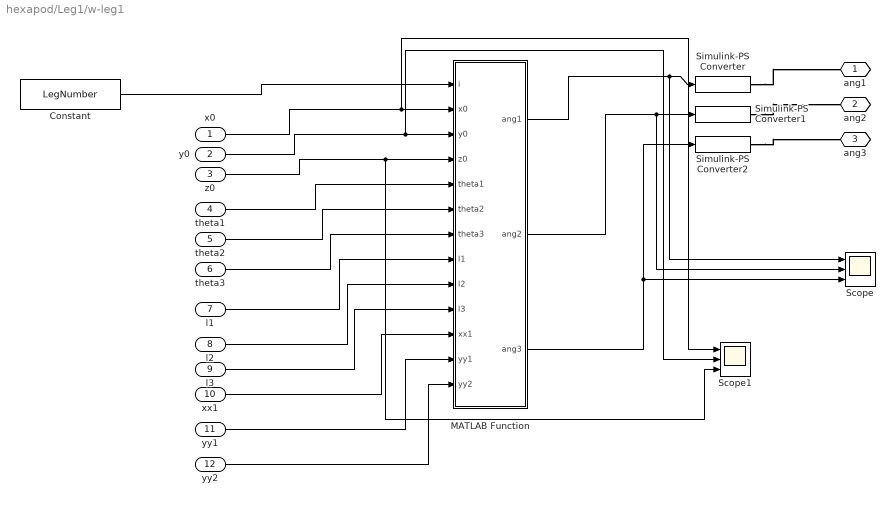
== system hexapod/Leg1/w-leg1 ==
  x0 : Inport
  y0 : Inport  Port=2
  z0 : Inport  Port=3
  theta1 : Inport  Port=4
  theta2 : Inport  Port=5
  theta3 : Inport  Port=6
  l1 : Inport  Port=7
  l2 : Inport  Port=8
  l3 : Inport  Port=9
  xx1 : Inport  Port=10
  yy1 : Inport  Port=11
  yy2 : Inport  Port=12
  Constant : Constant  Value=LegNumber
  MATLAB Function : MATLAB Function  TreatAsAtomicUnit=on
  Scope : Scope  NumInputPorts=3
  Scope1 : Scope  NumInputPorts=3
  Simulink-PS Converter : nesl_utility/Simulink-PS Converter  PhysicalDomain=network_engine_domain  SubClassName=ps_input  LeftPortType=input  RightPortType=output  PseudoPeriodic=off  Frequencies=[]  NoiseDistribution=none  NoiseParameters=[]  Unit=1  AffineConversion=off  FilteringAndDerivatives=filter  SimscapeFilterOrder=2  InputFilterTimeConstant=0.001  UdotUserProvided=0
      settings: SourceProductBaseCode=SS,PW,VE
  Simulink-PS Converter1 : nesl_utility/Simulink-PS Converter  PhysicalDomain=network_engine_domain  SubClassName=ps_input  LeftPortType=input  RightPortType=output  PseudoPeriodic=off  Frequencies=[]  NoiseDistribution=none  NoiseParameters=[]  Unit=1  AffineConversion=off  FilteringAndDerivatives=filter  SimscapeFilterOrder=2  InputFilterTimeConstant=0.001  UdotUserProvided=0
      settings: SourceProductBaseCode=SS,PW,VE
  Simulink-PS Converter2 : nesl_utility/Simulink-PS Converter  PhysicalDomain=network_engine_domain  SubClassName=ps_input  LeftPortType=input  RightPortType=output  PseudoPeriodic=off  Frequencies=[]  NoiseDistribution=none  NoiseParameters=[]  Unit=1  AffineConversion=off  FilteringAndDerivatives=filter  SimscapeFilterOrder=2  InputFilterTimeConstant=0.001  UdotUserProvided=0
      settings: SourceProductBaseCode=SS,PW,VE
  ang1 : PMIOPort  Side=Right
  ang2 : PMIOPort  Port=2  Side=Right
  ang3 : PMIOPort  Port=3  Side=Right
  wires:
  yy2/1 -> MATLAB Function/13(yy2)
  yy1/1 -> MATLAB Function/12(yy1)
  xx1/1 -> MATLAB Function/11(xx1)
  x0/1 -> MATLAB Function/2(x0), Scope1/1
  z0/1 -> MATLAB Function/4(z0), Scope1/3
  MATLAB Function/1(ang1) -> Simulink-PS Converter/1, Scope/1
  Constant/1 -> MATLAB Function/1(i)
  y0/1 -> MATLAB Function/3(y0), Scope1/2
  MATLAB Function/2(ang2) -> Simulink-PS Converter1/1, Scope/2
  MATLAB Function/3(ang3) -> Scope/3, Simulink-PS Converter2/1
  theta1/1 -> MATLAB Function/5(theta1)
  theta2/1 -> MATLAB Function/6(theta2)
  theta3/1 -> MATLAB Function/7(theta3)
  l1/1 -> MATLAB Function/8(l1)
  l2/1 -> MATLAB Function/9(l2)
  l3/1 -> MATLAB Function/10(l3)
  connections:
  Simulink-PS Converter2/RConn1 -- ang3/RConn1
  Simulink-PS Converter1/RConn1 -- ang2/RConn1
  Simulink-PS Converter/RConn1 -- ang1/RConn1

== system hexapod/Leg2/leg1 ==
  Revolute Joint : sm_lib/Joints/Revolute Joint  JointMode=Normal  SenseConstraintForce=off  SenseConstraintForceX=off  SenseConstraintForceY=off  SenseConstraintForceZ=off  SenseConstraintTorque=off  SenseConstraintTorqueX=off  SenseConstraintTorqueY=off  SenseConstraintTorqueZ=off  SenseTotalForce=off  SenseTotalForceX=off  SenseTotalForceY=off  SenseTotalForceZ=off  SenseTotalTorque=off  SenseTotalTorqueX=off  SenseTotalTorqueY=off  SenseTotalTorqueZ=off  CompositeWrenchDir=FollowerOnBase  CompositeWrenchFrame=BaseFrame  EquilibriumPosition=0  EquilibriumPositionUnits=deg  SpringStiffness=0  SpringStiffnessUnits=N*m/deg  DampingCoefficient=0  DampingCoefficientUnits=N*m/(deg/s)  TorqueActuationMode=ComputedTorque  MotionActuationMode=InputMotion  SensePosition=off  SenseVelocity=off  SenseAcceleration=off  SenseTorqueForce=off  SenseLowerLimitTorqueForce=off  SenseUpperLimitTorqueForce=off  LowerLimitSpecify=off  LowerLimitBound=-90  LowerLimitBoundUnits=deg  LowerLimitStiffness=1e4  LowerLimitStiffnessUnits=N*m/deg  LowerLimitDamping=10  LowerLimitDampingUnits=N*m/(deg/s)  LowerLimitTransitionRegionWidth=0.1  LowerLimitTransitionRegionWidthUnits=deg  UpperLimitSpecify=off  UpperLimitBound=90  UpperLimitBoundUnits=deg  UpperLimitStiffness=1e4  UpperLimitStiffnessUnits=N*m/deg  UpperLimitDamping=10  UpperLimitDampingUnits=N*m/(deg/s)  UpperLimitTransitionRegionWidth=0.1  UpperLimitTransitionRegionWidthUnits=deg  PositionTargetSpecify=off  PositionTargetPriority=High  PositionTargetValue=0  PositionTargetValueUnits=deg  VelocityTargetSpecify=off  VelocityTargetPriority=High  VelocityTargetValue=0  VelocityTargetValueUnits=deg/s
  Revolute Joint1 : sm_lib/Joints/Revolute Joint  JointMode=Normal  SenseConstraintForce=off  SenseConstraintForceX=off  SenseConstraintForceY=off  SenseConstraintForceZ=off  SenseConstraintTorque=off  SenseConstraintTorqueX=off  SenseConstraintTorqueY=off  SenseConstraintTorqueZ=off  SenseTotalForce=off  SenseTotalForceX=off  SenseTotalForceY=off  SenseTotalForceZ=off  SenseTotalTorque=off  SenseTotalTorqueX=off  SenseTotalTorqueY=off  SenseTotalTorqueZ=off  CompositeWrenchDir=FollowerOnBase  CompositeWrenchFrame=BaseFrame  EquilibriumPosition=0  EquilibriumPositionUnits=deg  SpringStiffness=0  SpringStiffnessUnits=N*m/deg  DampingCoefficient=0  DampingCoefficientUnits=N*m/(deg/s)  TorqueActuationMode=ComputedTorque  MotionActuationMode=InputMotion  SensePosition=off  SenseVelocity=off  SenseAcceleration=off  SenseTorqueForce=off  SenseLowerLimitTorqueForce=off  SenseUpperLimitTorqueForce=off  LowerLimitSpecify=off  LowerLimitBound=-90  LowerLimitBoundUnits=deg  LowerLimitStiffness=1e4  LowerLimitStiffnessUnits=N*m/deg  LowerLimitDamping=10  LowerLimitDampingUnits=N*m/(deg/s)  LowerLimitTransitionRegionWidth=0.1  LowerLimitTransitionRegionWidthUnits=deg  UpperLimitSpecify=off  UpperLimitBound=90  UpperLimitBoundUnits=deg  UpperLimitStiffness=1e4  UpperLimitStiffnessUnits=N*m/deg  UpperLimitDamping=10  UpperLimitDampingUnits=N*m/(deg/s)  UpperLimitTransitionRegionWidth=0.1  UpperLimitTransitionRegionWidthUnits=deg  PositionTargetSpecify=off  PositionTargetPriority=High  PositionTargetValue=0  PositionTargetValueUnits=deg  VelocityTargetSpecify=off  VelocityTargetPriority=High  VelocityTargetValue=0  VelocityTargetValueUnits=deg/s
  Revolute Joint2 : sm_lib/Joints/Revolute Joint  JointMode=Normal  SenseConstraintForce=off  SenseConstraintForceX=off  SenseConstraintForceY=off  SenseConstraintForceZ=off  SenseConstraintTorque=off  SenseConstraintTorqueX=off  SenseConstraintTorqueY=off  SenseConstraintTorqueZ=off  SenseTotalForce=off  SenseTotalForceX=off  SenseTotalForceY=off  SenseTotalForceZ=off  SenseTotalTorque=off  SenseTotalTorqueX=off  SenseTotalTorqueY=off  SenseTotalTorqueZ=off  CompositeWrenchDir=FollowerOnBase  CompositeWrenchFrame=BaseFrame  EquilibriumPosition=0  EquilibriumPositionUnits=deg  SpringStiffness=0  SpringStiffnessUnits=N*m/deg  DampingCoefficient=0  DampingCoefficientUnits=N*m/(deg/s)  TorqueActuationMode=ComputedTorque  MotionActuationMode=InputMotion  SensePosition=off  SenseVelocity=off  SenseAcceleration=off  SenseTorqueForce=off  SenseLowerLimitTorqueForce=off  SenseUpperLimitTorqueForce=off  LowerLimitSpecify=off  LowerLimitBound=-90  LowerLimitBoundUnits=deg  LowerLimitStiffness=1e4  LowerLimitStiffnessUnits=N*m/deg  LowerLimitDamping=10  LowerLimitDampingUnits=N*m/(deg/s)  LowerLimitTransitionRegionWidth=0.1  LowerLimitTransitionRegionWidthUnits=deg  UpperLimitSpecify=off  UpperLimitBound=90  UpperLimitBoundUnits=deg  UpperLimitStiffness=1e4  UpperLimitStiffnessUnits=N*m/deg  UpperLimitDamping=10  UpperLimitDampingUnits=N*m/(deg/s)  UpperLimitTransitionRegionWidth=0.1  UpperLimitTransitionRegionWidthUnits=deg  PositionTargetSpecify=off  PositionTargetPriority=High  PositionTargetValue=0  PositionTargetValueUnits=deg  VelocityTargetSpecify=off  VelocityTargetPriority=High  VelocityTargetValue=0  VelocityTargetValueUnits=deg/s
  link1 : Subsystem
  link2 : Subsystem
  link3 : Subsystem
  base : PMIOPort  Side=Left
  ang1 : PMIOPort  Port=2  Side=Left
  ang2 : PMIOPort  Port=3  Side=Left
  ang3 : PMIOPort  Port=4  Side=Left
  end : PMIOPort  Port=5  Side=Right
  connections:
  Revolute Joint1/LConn2 -- ang2/RConn1
  base/RConn1 -- Revolute Joint/LConn1
  end/RConn1 -- link3/RConn1
  Revolute Joint2/LConn1 -- link2/RConn1
  link2/LConn1 -- Revolute Joint1/RConn1
  Revolute Joint1/LConn1 -- link1/RConn1
  Revolute Joint2/RConn1 -- link3/LConn1
  Revolute Joint/RConn1 -- link1/LConn1
  Revolute Joint/LConn2 -- ang1/RConn1
  Revolute Joint2/LConn2 -- ang3/RConn1
